simulink model "MicrogridControl"  (R2025b)
settings: Solver=VariableStepAuto  StartTime=0.0  StopTime=8  FixedStep=Ts  RelTol=1e-3
PreLoadFcn:
  | NormalOperation;
  | MicrogridControlParam;
undefined symbols (not defined in the file): base, bessModeInitial, bessSystem, bessVoltage, breakerStatus, DiscIntNeverNeededParam, ee_sli_rtmsupport, event, gcbh, generator, gflInverter, gfmInverter, Inertia, lineInductance, lineResistance, machine, plannedIsland, pmsm, powerLimit, powerQuality, PV, PVInverter, ref, resync, solar, solarInsolationChange, systemFrequency, Ts, windController, windSystem, windTurbine
libraries: nesl_utility x234, ee_lib x174, fl_lib x143, eeGeneralControl x137, simulink x78, eeTransforms x47, slpidlib x23, nesl_utility_internal x12, eePwmGenerator x9, eeSinusoidalMeasurementV2 x9, custom_lib x7, batteryecm_lib x6
(part 15 of 25)

== system MicrogridControl/BESS/BESS Integrated/Detailed/BESS Controller/Grid Forming/VoltageCurrentControl ==
  In Bus Element : Inport  PortName=currentLimiting  Element=Vmd
  In Bus Element1 : Inport  PortName=currentLimiting  Element=Vmq
  In Bus Element6 : Inport  PortName=currentLimiting  Element=Idmax
  In Bus Element7 : Inport  PortName=currentLimiting  Element=Iqmax
  Bus Element In6 : Inport  Port=2  PortName=activeControl  Element=w
  Bus Element In1 : Inport  Port=2  PortName=activeControl  Element=angle
  Reset : Inport  Port=3
  In Bus Element2 : Inport  Port=4  PortName=measure  Element=Vgd
  In Bus Element3 : Inport  Port=4  PortName=measure  Element=Vgq
  In Bus Element4 : Inport  Port=4  PortName=measure  Element=Igd
  In Bus Element5 : Inport  Port=4  PortName=measure  Element=Igq
  Controller : Subsystem
      settings: PortSchema="{\"entries\":[{\"content\":{\"sides\":[{\"content\":{\"connectorIds\":[\"In1\",\"In2\",\"In3\",\"In4\",\"In5\",\"In6\",\"In7\",\"In8\",\"In9\"]},\"type\":\"ConnectorPlacement.EquallySpacedRectSide\",\"uuid\":\"29d30ab3-0ae0-4ae6-aaee-46c6f5faca9c\"},{\"content\":{\"connectorIds\":[\"Out1\",\"Out2\"],\"side\":\"RIGHT\"},\"type\":\"ConnectorPlacement.EquallySpacedRectSide\",\"uuid\":\"4918c3a7-9f8f-4af5-ac25-a0a0710917b2\"},{\"content\":{\"connectorIds\":[\"In10\"],\"side\":\"TOP\"},\"type\":\"ConnectorPlacement.EquallySpacedRectSide\",\"uuid\":\"c6ee8000-0a39-46c2-b8e8-8b73a56a82d9\"}]},\"type\":\"ConnectorPlacement.EquallySpacedConnector\",\"uuid\":\"193e0bc8-3764-41d1-9278-3938c4a9e9f5\"}],\"packageUris\":[\"http://schema.mathworks.com/mf0/Connector/R2020b\"],\"version\":\"1.0\"}"
  Modulation Signal : Subsystem
  mabc : Outport
  wires:
  Reset/1 -> Controller/10(Reset)
  Bus Element In1/1 -> Modulation Signal/3(Angle)
  In Bus Element1/1 -> Controller/3(Vgqref)
  In Bus Element/1 -> Controller/2(Vgdref)
  Bus Element In6/1 -> Controller/1(Angfreq)
  In Bus Element3/1 -> Controller/5(Vsq)
  In Bus Element2/1 -> Controller/4(Vsd)
  In Bus Element7/1 -> Controller/9(Iqmax)
  In Bus Element6/1 -> Controller/8(Idmax)
  In Bus Element5/1 -> Controller/7(Iq)
  In Bus Element4/1 -> Controller/6(Id)
  Controller/1(Vd) -> Modulation Signal/1(Vd)
  Modulation Signal/1(mabc) -> mabc/1
  Controller/2(Vq) -> Modulation Signal/2(Vq)

== system MicrogridControl/BESS/BESS Integrated/Detailed/BESS Plant/Converter/Average ==
  mabc : Inport
  Converter : ee_lib/Semiconductors & Converters/Converters/Average-Value Voltage Source Converter (Three-Phase)  port_option=ee.enum.threePhasePort.composite  frequency_option=ee.enum.converters.frequency.variable  input_option=ee.enum.converters.inputOption.ModWave  FRated=60 Hz  losses_parameterization=ee.enum.converters.losses.fixed  Pfixed=0.5 W  ks=0.01  kc1=1.7 V  kc2=0.01 Ohm  Ploss_vect=[100, 800, 1870, 3250, 4900] W  Irms_vect=[10, 100, 200, 300, 400] A  Vdc_nom=300 V  thermal_mass=30000 J/K  temperature_specify=off  temperature_priority=High  temperature=298.15 K  temperature_nominal_specify=off  temperature_nominal_value=1  temperature_nominal_unit=K
      settings: InternalSimscapePortConfiguration="{\"Bottom\":[],\"Left\":[{\"id\":\"ModWave\",\"label\":\"ModWave\",\"type\":\"input\"},{\"id\":\"N\",\"label\":\"~\",\"type\":\"foundation.electrical.three_phase\"}],\"Right\":[{\"id\":\"p\",\"label\":\"+\",\"type\":\"foundation.electrical.electrical\"},{\"id\":\"n\",\"label\":\"-\",\"type\":\"foundation.electrical.electrical\"}],\"Top\":[]}"
  Simulink-PS Converter : nesl_utility/Simulink-PS Converter  PhysicalDomain=network_engine_domain  SubClassName=ps_input  LeftPortType=input  RightPortType=output  PseudoPeriodic=off  Frequencies=[]  NoiseDistribution=none  NoiseParameters=[]  Unit=1  AffineConversion=off  FilteringAndDerivatives=provide  SimscapeFilterOrder=1  InputFilterTimeConstant=0.001  UdotUserProvided=0
  + : PMIOPort  Side=Left
  - : PMIOPort  Port=2  Side=Left
  ~ : PMIOPort  Port=3  Side=Right
  wires:
  mabc/1 -> Simulink-PS Converter/1
  connections:
  Simulink-PS Converter/RConn1 -- Converter/LConn1
  ~/RConn1 -- Converter/LConn2
  -/RConn1 -- Converter/RConn2
  +/RConn1 -- Converter/RConn1

== system MicrogridControl/BESS/BESS Integrated/Detailed/BESS Plant/Converter/Switching ==
  mabc : Inport
  Add : Sum
  Constant1 : Constant
  Converter : ee_lib/Semiconductors & Converters/Converters/Converter (Three-Phase)  port_option=ee.enum.threePhasePort.composite  fidelity_option=ee.enum.converters.fidelity.detailed  device_type=ee.enum.converters.switchingdevice.ideal  showThermalPort=false  K=0  Vth=1 V  Vgt=1 V  Vgt_off=-1 V  Ih=1 A  Vf=0.8 V  Ron=0.001 Ohm  Rds=0.001 Ohm  Goff=1e-6 1/Ohm  Eon_scalar=22.86e-3 J  Eoff_scalar=17.14e-3 J  Eoff_natural_commutation=10e-3 J  Voff=300 V  Iout_scalar=600 A  onCurrentMeasDelay=0 s  useCurrentFromPreviousCycle=false  useVoltageFromPreviousCycle=false  diode_param=ee.enum.converters.protectiondiode.nodynamics  diode_Vf=0.01 V  diode_Ron=0.0001 Ohm  diode_Goff=1e-5 1/Ohm  diode_C=50 nF  diode_iRM=-235 A  diode_iF=300 A  diode_idot=-50 A/us  diode_trr_param=ee.enum.converters.diodetrr.trr_factor  diode_trr_factor=3  diode_trr=15 us  diode_Qrr=1500 s*uA  diode_rec_loss_model=ee.enum.diode.reverseRecoveryModel.fixed  diode_ErecVal=0 J  diode_scaleWithIandV=false  diode_ErecMat=zeros(2, 3) J  diode_TjrecVec=[298.15, 398.15] K  diode_IfrecVec=[.1, 1, 10] A  diode_IrecVal=10 A  diode_VrecVal=10 V  diode_tFilter=1 / 1000 / 100 s  thermal_network_parameterization=ee.enum.thermalNetworkTopology.external  Rth=[.08, .5] K/W  Rth_Cauer=[.08, .1, .5] K/W  Rth_Foster=[.08, .14, .22, .16] K/W  thermal_mass_parameterization=ee.enum.thermalNetwork.timeconstant  thermal_mass=[.01, .5] J/K  thermal_mass_Cauer=[.01, .1, .5] J/K  thermal_mass_Foster=[.001, .005, .05, .5] J/K  thermal_time_constant=[.001, .2] s  thermal_time_constant_Cauer=[.001, .1, .2] s  thermal_time_constant_Foster=[7e-05, .0007, .01, .08] s  thermal_mass_initial_temperatures=[25, 25] degC  thermal_mass_initial_temperatures_Cauer=[25, 25, 25] degC  junction_thermal_mass=0.01 J/K  Tvec_initial_Foster=[25, 25, 25, 25] degC  snubber_type=ee.enum.converters.snubber.exclude  Cs=1e-7 F  Rs=0.1 Ohm  Vce_loss=[0, 150, 300] V
  Demux : Demux  Outputs=3
  Demux1 : Demux  Outputs=3
  Gain : Gain  Gain=5
  Gain1 : Gain  Gain=0.5
  PWM Generator : eePwmGenerator/PWM Generator  CarrCount=Up  Tper=1/(fSw*1000)  Tdelay=0  Ts=1/(10*fSw*1000)
  Pulse Generation : Subsystem
  Rate Transition1 : RateTransition  OutPortSampleTime=1/(10*fSw*1000)
  Simulink-PS Converter{1..6} (6 alike) : nesl_utility/Simulink-PS Converter  PhysicalDomain=network_engine_domain  SubClassName=ps_input  LeftPortType=input  RightPortType=output  PseudoPeriodic=off  Frequencies=[]  NoiseDistribution=none  NoiseParameters=[]  Unit=1  AffineConversion=off  FilteringAndDerivatives=provide  SimscapeFilterOrder=1  InputFilterTimeConstant=0.001  UdotUserProvided=0
  Six-Pulse Gate Multiplexer : ee_lib/Semiconductors & Converters/Converters/Six-Pulse Gate Multiplexer  port_option=ee.enum.controlport.ps
  + : PMIOPort  Side=Left
  ~ : PMIOPort  Port=2  Side=Right
  - : PMIOPort  Port=3  Side=Left
  wires:
  Demux1/1 -> [AL]
  [BL] -> Simulink-PS Converter3/1
  [AH] -> Simulink-PS Converter6/1
  Demux1/3 -> [CL]
  Gain1/1 -> Rate Transition1/1
  Demux/3 -> [CH]
  Demux/2 -> [BH]
  [CL] -> Simulink-PS Converter1/1
  Constant1/1 -> Add/2
  Add/1 -> Gain1/1
  Gain/1 -> Pulse Generation/1(G)
  PWM Generator/1 -> Gain/1
  mabc/1 -> Add/1
  [CH] -> Simulink-PS Converter2/1
  [AL] -> Simulink-PS Converter5/1
  Demux1/2 -> [BL]
  Demux/1 -> [AH]
  Rate Transition1/1 -> PWM Generator/1
  Pulse Generation/2(G2) -> Demux1/1
  Pulse Generation/1(G1) -> Demux/1
  [BH] -> Simulink-PS Converter4/1
  connections:
  ~/RConn1 -- Converter/LConn2
  Six-Pulse Gate Multiplexer/LConn2 -- Simulink-PS Converter5/RConn1
  Simulink-PS Converter2/RConn1 -- Six-Pulse Gate Multiplexer/LConn5
  Simulink-PS Converter1/RConn1 -- Six-Pulse Gate Multiplexer/LConn6
  Six-Pulse Gate Multiplexer/LConn3 -- Simulink-PS Converter4/RConn1
  Six-Pulse Gate Multiplexer/RConn1 -- Converter/LConn1
  Six-Pulse Gate Multiplexer/LConn1 -- Simulink-PS Converter6/RConn1
  Six-Pulse Gate Multiplexer/LConn4 -- Simulink-PS Converter3/RConn1
  +/RConn1 -- Converter/RConn1
  -/RConn1 -- Converter/RConn2

== system MicrogridControl/BESS/BESS Integrated/Detailed/Filter & Measurements/PLL & Measurements/Measurement1 ==
  u : Inport
  Lead-Lag (Discrete or Continuous) : eeGeneralControl/Lead-Lag (Discrete or Continuous)  T1=0  T2=1e-3  B=inf  A=-inf  init_option=Inherited from block input  x0=0  Ts=Ts
  Vg : Outport
  wires:
  u/1 -> Lead-Lag (Discrete or Continuous)/1
  Lead-Lag (Discrete or Continuous)/1 -> Vg/1

== system MicrogridControl/BESS/BESS Integrated/Detailed/Filter & Measurements/PLL & Measurements/Measurement2 ==
  u : Inport
  Lead-Lag (Discrete or Continuous) : eeGeneralControl/Lead-Lag (Discrete or Continuous)  T1=0  T2=1e-3  B=inf  A=-inf  init_option=Inherited from block input  x0=0  Ts=Ts
  Vg : Outport
  wires:
  u/1 -> Lead-Lag (Discrete or Continuous)/1
  Lead-Lag (Discrete or Continuous)/1 -> Vg/1

== system MicrogridControl/BESS/BESS Integrated/Detailed/Filter & Measurements/PLL & Measurements/Subsystem ==
  Vabc : Inport
  Iabc : Inport  Port=2
  Demux : Demux  Outputs=3
  Demux1 : Demux  Outputs=3
  Park Transform : eeTransforms/Park Transform  AxisAlignment=Q-axis  PowerInvariant=off
  Park Transform1 : eeTransforms/Park Transform  AxisAlignment=Q-axis  PowerInvariant=off
  Scope : Scope  NumInputPorts=2
      settings: ActiveDisplayYMinimum=0.95416  ActiveDisplayYMaximum=1.02793  DataLoggingVariableName=ScopeData5
  Scope1 : Scope  NumInputPorts=2
      settings: ActiveDisplayYMinimum=-2.7903298017751648  ActiveDisplayYMaximum=-1.7770998587100291  DataLoggingVariableName=ScopeData10
  "Sinusoidal Measurement (PLL, Three-Phase)" : eeSinusoidalMeasurementV2/Sinusoidal Measurement (PLL, Three-Phase)  InputFilter=on  InputNormalization=off  Kp_LF=40  Ki_LF=1000  F0=frequency  Theta0=0  Ts=Ts
  Terminator : Terminator
  Terminator1 : Terminator
  mag : Outport
  freq : Outport  Port=2
  angle : Outport  Port=3
  Vd : Outport  Port=4
  Vq : Outport  Port=5
  Id1 : Outport  Port=6
  Iq1 : Outport  Port=7
  wires:
  Iabc/1 -> Park Transform1/1
  Demux1/3 -> Terminator1/1
  Demux1/2 -> Scope1/2, Iq1/1
  Demux1/1 -> Scope1/1, Id1/1
  Park Transform1/1 -> Demux1/1
  "Sinusoidal Measurement (PLL, Three-Phase)"/3 -> mag/1
  "Sinusoidal Measurement (PLL, Three-Phase)"/1 -> freq/1
  "Sinusoidal Measurement (PLL, Three-Phase)"/2 -> Park Transform/2, Park Transform1/2, angle/1
  Demux/2 -> Vq/1, Scope/2
  Demux/1 -> Vd/1, Scope/1
  Park Transform/1 -> Demux/1
  Vabc/1 -> "Sinusoidal Measurement (PLL, Three-Phase)"/1, Park Transform/1
  Demux/3 -> Terminator/1

== system MicrogridControl/BESS/BESS Integrated/Simplified/Grid Forming/Reference Generator/If Action Subsystem ==
  PRef : Inport
  P : Inport  Port=2
  QRef : Inport  Port=3
  Q : Inport  Port=4
  Action Port : ActionPort
  Add : Sum  Inputs=-+
  Add1 : Sum  Inputs=+-
  Add2 : Sum
  Add3 : Sum  Inputs=+-
  Add4 : Sum  Inputs=-+
  Constant : Constant  Value=2*pi*frequency  SampleTime=-1
  Constant2 : Constant
  Constant3 : Constant
  Gain : Gain  Gain=activeDroop
  Gain1 : Gain  Gain=reactiveDroop
  Gain4 : Gain  Gain=Vac
  Gain5 : Gain  Gain=2*pi*frequency
  Integrator with Wrapped State (Discrete or Continuous) : eeGeneralControl/Integrator with Wrapped State (Discrete or Continuous)  LabelModeActiveChoice=Discrete  WrappedStateUpperValue=2*pi  WrappedStateLowerValue=0  x0=0  Ts=-1
  Integrator with Wrapped State (Discrete or Continuous)1 : eeGeneralControl/Integrator with Wrapped State (Discrete or Continuous)  LabelModeActiveChoice=Discrete  WrappedStateUpperValue=2*pi  WrappedStateLowerValue=0  x0=0  Ts=-1
  Saturation : Saturate  UpperLimit=1.1  LowerLimit=0.9
  Scope : Scope
      settings: ActiveDisplayYMinimum=-1  ActiveDisplayYMaximum=1  DataLoggingVariableName=ScopeData2
  Scope1 : Scope
      settings: ActiveDisplayYMinimum=-1  ActiveDisplayYMaximum=1  DataLoggingVariableName=ScopeData3
  Scope2 : Scope  NumInputPorts=2
      settings: ActiveDisplayYMinimum=-1  ActiveDisplayYMaximum=1
  Scope3 : Scope  NumInputPorts=2
      settings: ActiveDisplayYMinimum=-1  ActiveDisplayYMaximum=1  DataLoggingVariableName=ScopeData2
  Vt : Outport
  Ph : Outport  Port=2
  wires:
  Add4/1 -> Scope/1, Gain5/1
  Gain/1 -> Add4/1
  Add1/1 -> Gain1/1
  Add2/1 -> Scope1/1, Saturation/1
  Gain5/1 -> Integrator with Wrapped State (Discrete or Continuous)/1
  Constant3/1 -> Add4/2
  Integrator with Wrapped State (Discrete or Continuous)/1 -> Add3/1
  Constant2/1 -> Add2/2
  Gain1/1 -> Add2/1
  Gain4/1 -> Vt/1
  QRef/1 -> Add1/1, Scope2/1
  Saturation/1 -> Gain4/1
  Add/1 -> Gain/1
  PRef/1 -> Add/1, Scope3/1
  Add3/1 -> Ph/1
  Constant/1 -> Integrator with Wrapped State (Discrete or Continuous)1/1
  Integrator with Wrapped State (Discrete or Continuous)1/1 -> Add3/2
  P/1 -> Add/2, Scope3/2
  Q/1 -> Add1/2, Scope2/2

== system MicrogridControl/BESS/BESS Integrated/Simplified/Grid Forming/Reference Generator/If Action Subsystem1 ==
  PRef : Inport
  P : Inport  Port=2
  VRef : Inport  Port=3
  V : Inport  Port=4
  Action Port : ActionPort
  Add : Sum  Inputs=+-
  Add1 : Sum  Inputs=+-
  Add2 : Sum
  Add3 : Sum  Inputs=+-
  Add4 : Sum  Inputs=-+
  Constant2 : Constant
  Constant3 : Constant
  Constant4 : Constant  Value=0
  Gain : Gain  Gain=reactiveDroop
  Gain1 : Gain  Gain=activeDroop
  Gain4 : Gain  Gain=systemVoltage
  Gain5 : Gain  Gain=2*pi*systemFrequency
  Integrator with Wrapped State (Discrete or Continuous) : eeGeneralControl/Integrator with Wrapped State (Discrete or Continuous)  LabelModeActiveChoice=Discrete  WrappedStateUpperValue=2*pi  WrappedStateLowerValue=0  x0=0  Ts=-1
  Saturation : Saturate  UpperLimit=1.1  LowerLimit=0.9
  Vt : Outport
  Ph : Outport  Port=2
  wires:
  Add/1 -> Gain/1
  Constant4/1 -> Add3/2
  Add4/1 -> Gain5/1
  Gain/1 -> Add4/1
  Add1/1 -> Gain1/1
  Add2/1 -> Saturation/1
  Gain5/1 -> Integrator with Wrapped State (Discrete or Continuous)/1
  Constant3/1 -> Add4/2
  Integrator with Wrapped State (Discrete or Continuous)/1 -> Add3/1
  Constant2/1 -> Add2/2
  Gain1/1 -> Add2/1
  V/1 -> Add/2
  Gain4/1 -> Vt/1
  P/1 -> Add1/2
  VRef/1 -> Add/1
  PRef/1 -> Add1/1
  Add3/1 -> Ph/1
  Saturation/1 -> Gain4/1

== system MicrogridControl/BESS/BESS Integrated1/Detailed/BESS Controller/Grid Following/Current_controller ==
  id-ref : Inport
  ipvd : Inport  Port=2
  iqref : Inport  Port=3
  iq : Inport  Port=4
  Vd : Inport  Port=5
  Vq : Inport  Port=6
  Constant4 : Constant  Value=0
  Gain1 : Gain  Gain=2*1*pi*frequency*L/zbase
  Gain2 : Gain  Gain=2*1*pi*frequency*L/zbase
  Mux1 : Mux  Inputs=3
  PID Controller : slpidlib/PID Controller  Controller=PID  Form=Parallel  TimeDomain=Discrete-time  UseExternalTs=off  SampleTime=-1  IntegratorMethod=Forward Euler  FilterMethod=Forward Euler  ControllerParametersSource=internal  P=Kpic  I=Kiic  UseKiTs=off  D=Kd  UseExternalDerivativeSource=off  N=100  UseFilter=on  TunerSelectOption=Transfer Function Based (PID Tuner App)  InitialConditionSource=internal  InitialConditionForIntegrator=0  InitialConditionForFilter=0  DifferentiatorICPrevScaledInput=0  ExternalReset=none  TrackingMode=off  Kt=1  LimitOutput=off  SatLimitsSource=internal  UpperSaturationLimit=inf  LowerSaturationLimit=-inf  LinearizeAsGain=on  AntiWindupMode=none  Kb=1  LimitIntegrator=off  UpperIntegratorSaturationLimit=inf  LowerIntegratorSaturationLimit=-inf  POutMin=[]  POutMax=[]  IOutMin=[]  IOutMax=[]  DOutMin=[]  DOutMax=[]  NOutMin=[]  NOutMax=[]  SumOutMin=[]  SumOutMax=[]  SaturationOutMin=[]  SaturationOutMax=[]  PParamMin=[]  PParamMax=[]  IParamMin=[]  IParamMax=[]  DParamMin=[]  DParamMax=[]  NParamMin=[]  NParamMax=[]  KbParamMin=[]  KbParamMax=[]  KtParamMin=[]  KtParamMax=[]  KbOutMin=[]  KbOutMax=[]  KtOutMin=[]  KtOutMax=[]  IntegratorOutMin=[]  IntegratorOutMax=[]  FilterOutMin=[]  FilterOutMax=[]  SumI1OutMin=[]  SumI1OutMax=[]  SumI2OutMin=[]  SumI2OutMax=[]  SumI3OutMin=[]  SumI3OutMax=[]  SumI4OutMin=[]  SumI4OutMax=[]  SumDOutMin=[]  SumDOutMax=[]  DifferentiatorOutMin=[]  DifferentiatorOutMax=[]  FilterDiffOutCoefMin=[]  FilterDiffOutCoefMax=[]  ReciprocalOutMin=[]  ReciprocalOutMax=[]  SumDenOutMin=[]  SumDenOutMax=[]  SumNumOutMin=[]  SumNumOutMax=[]  DivideOutMin=[]  DivideOutMax=[]  UdiffTsProdOutMin=[]  UdiffTsProdOutMax=[]  NTsProdOutMin=[]  NTsProdOutMax=[]  UintegralTsProdOutMin=[]  UintegralTsProdOutMax=[]  UngainTsProdOutMin=[]  UngainTsProdOutMax=[]  ClampingZeroOutDataTypeStr=Inherit: Inherit via back propagation  ClampingZeroOutMin=[]  ClampingZeroOutMax=[]  FilterDenConstantOutDataTypeStr=Inherit: Inherit via back propagation  FilterDenConstantOutMin=[]  FilterDenConstantOutMax=[]  PCopyOutDataTypeStr=Inherit: Inherit via back propagation  PCopyOutMin=[]  PCopyOutMax=[]  NCopyOutDataTypeStr=Inherit: Inherit via back propagation  NCopyOutMin=[]  NCopyOutMax=[]  IntegratorContinuousStateAttributes=''  IntegratorStateMustResolveToSignalObject=off  IntegratorRTWStateStorageClass=Auto  FilterContinuousStateAttributes=''  FilterStateMustResolveToSignalObject=off  FilterRTWStateStorageClass=Auto  ParallelPVariant=InternalParameters  IdealPVariant=Disabled  IVariant=InternalParameters  DVariant=InternalParameters  IntegratorVariant=Discrete  SatVariant=Disabled  AWVariant=Passthrough  PCopyVariant=Disabled  TRVariant=Disabled  FdbkBlocksVariant=Forward  IdealPFdbkVariant=Disabled  SatFdbkVariant=Disabled  DerivativeFilterVariant=ForwardEulerFilter  NVariant=InternalParameters  NCopyVariant=Disabled  FilterICVariant=InternalICsFilter  IntegratorICVariant=InternalICs  ExternalResetVariant=Disabled  TRSumVariant=Passthrough  SumFdbkVariant=Disabled  SumVariant=Sum_PID  TsampFilterVariant=InternalTs  TsampNgainVariant=Passthrough  TsampIntegralVariant=Disabled_SignalSpec  ExternalSaturationOutDataTypeStr=Inherit: Same as second input  DerivativeSourceVariant=ErrorSignal  PreIntVariant=InternalPreInt
  PID Controller1 : slpidlib/PID Controller  Controller=PID  Form=Parallel  TimeDomain=Discrete-time  UseExternalTs=off  SampleTime=-1  IntegratorMethod=Forward Euler  FilterMethod=Forward Euler  ControllerParametersSource=internal  P=Kpic  I=Kiic  UseKiTs=off  D=Kd  UseExternalDerivativeSource=off  N=100  UseFilter=on  TunerSelectOption=Transfer Function Based (PID Tuner App)  InitialConditionSource=internal  InitialConditionForIntegrator=0  InitialConditionForFilter=0  DifferentiatorICPrevScaledInput=0  ExternalReset=none  TrackingMode=off  Kt=1  LimitOutput=off  SatLimitsSource=internal  UpperSaturationLimit=inf  LowerSaturationLimit=-inf  LinearizeAsGain=on  AntiWindupMode=none  Kb=1  LimitIntegrator=off  UpperIntegratorSaturationLimit=inf  LowerIntegratorSaturationLimit=-inf  POutMin=[]  POutMax=[]  IOutMin=[]  IOutMax=[]  DOutMin=[]  DOutMax=[]  NOutMin=[]  NOutMax=[]  SumOutMin=[]  SumOutMax=[]  SaturationOutMin=[]  SaturationOutMax=[]  PParamMin=[]  PParamMax=[]  IParamMin=[]  IParamMax=[]  DParamMin=[]  DParamMax=[]  NParamMin=[]  NParamMax=[]  KbParamMin=[]  KbParamMax=[]  KtParamMin=[]  KtParamMax=[]  KbOutMin=[]  KbOutMax=[]  KtOutMin=[]  KtOutMax=[]  IntegratorOutMin=[]  IntegratorOutMax=[]  FilterOutMin=[]  FilterOutMax=[]  SumI1OutMin=[]  SumI1OutMax=[]  SumI2OutMin=[]  SumI2OutMax=[]  SumI3OutMin=[]  SumI3OutMax=[]  SumI4OutMin=[]  SumI4OutMax=[]  SumDOutMin=[]  SumDOutMax=[]  DifferentiatorOutMin=[]  DifferentiatorOutMax=[]  FilterDiffOutCoefMin=[]  FilterDiffOutCoefMax=[]  ReciprocalOutMin=[]  ReciprocalOutMax=[]  SumDenOutMin=[]  SumDenOutMax=[]  SumNumOutMin=[]  SumNumOutMax=[]  DivideOutMin=[]  DivideOutMax=[]  UdiffTsProdOutMin=[]  UdiffTsProdOutMax=[]  NTsProdOutMin=[]  NTsProdOutMax=[]  UintegralTsProdOutMin=[]  UintegralTsProdOutMax=[]  UngainTsProdOutMin=[]  UngainTsProdOutMax=[]  ClampingZeroOutDataTypeStr=Inherit: Inherit via back propagation  ClampingZeroOutMin=[]  ClampingZeroOutMax=[]  FilterDenConstantOutDataTypeStr=Inherit: Inherit via back propagation  FilterDenConstantOutMin=[]  FilterDenConstantOutMax=[]  PCopyOutDataTypeStr=Inherit: Inherit via back propagation  PCopyOutMin=[]  PCopyOutMax=[]  NCopyOutDataTypeStr=Inherit: Inherit via back propagation  NCopyOutMin=[]  NCopyOutMax=[]  IntegratorContinuousStateAttributes=''  IntegratorStateMustResolveToSignalObject=off  IntegratorRTWStateStorageClass=Auto  FilterContinuousStateAttributes=''  FilterStateMustResolveToSignalObject=off  FilterRTWStateStorageClass=Auto  ParallelPVariant=InternalParameters  IdealPVariant=Disabled  IVariant=InternalParameters  DVariant=InternalParameters  IntegratorVariant=Discrete  SatVariant=Disabled  AWVariant=Passthrough  PCopyVariant=Disabled  TRVariant=Disabled  FdbkBlocksVariant=Forward  IdealPFdbkVariant=Disabled  SatFdbkVariant=Disabled  DerivativeFilterVariant=ForwardEulerFilter  NVariant=InternalParameters  NCopyVariant=Disabled  FilterICVariant=InternalICsFilter  IntegratorICVariant=InternalICs  ExternalResetVariant=Disabled  TRSumVariant=Passthrough  SumFdbkVariant=Disabled  SumVariant=Sum_PID  TsampFilterVariant=InternalTs  TsampNgainVariant=Passthrough  TsampIntegralVariant=Disabled_SignalSpec  ExternalSaturationOutDataTypeStr=Inherit: Same as second input  DerivativeSourceVariant=ErrorSignal  PreIntVariant=InternalPreInt
  Scope : Scope  NumInputPorts=2
      settings: ActiveDisplayYMinimum=-1  ActiveDisplayYMaximum=1
  Scope1 : Scope  NumInputPorts=2
      settings: ActiveDisplayYMinimum=-1.21282  ActiveDisplayYMaximum=0.9154  DataLoggingVariableName=ScopeData2
  Sum1 : Sum  Inputs=|+-
  Sum3 : Sum  Inputs=|++-
  Sum4 : Sum  Inputs=|+++
  Sum5 : Sum  Inputs=|+-
  mdq0 : Outport
  wires:
  iqref/1 -> Sum5/1, Scope1/1
  Mux1/1 -> mdq0/1
  Sum4/1 -> [Eq], Mux1/2
  PID Controller1/1 -> Sum4/1
  Sum5/1 -> PID Controller1/1
  Constant4/1 -> Mux1/3
  Vd/1 -> Sum3/1
  Sum1/1 -> PID Controller/1
  iq/1 -> Sum5/2, Gain2/1, Scope1/2
  Vq/1 -> Sum4/2
  Gain1/1 -> Sum4/3
  id-ref/1 -> Sum1/1, Scope/1
  ipvd/1 -> Sum1/2, Gain1/1, Scope/2
  Gain2/1 -> Sum3/3
  Sum3/1 -> [Ed], Mux1/1
  PID Controller/1 -> Sum3/2

== system MicrogridControl/BESS/BESS Integrated1/Detailed/BESS Controller/Grid Following/Reference Current ==
  note: Avoid division by zero during start
  note: Current Limiters
  V_ref : Inport
  V-mag : Inport  Port=2
  del f : Inport  Port=3
  LVRT_iq : Inport  Port=4
  PRef : Inport  Port=5
  QRef : Inport  Port=6
  Constant1 : Constant
  Constant3 : Constant  Value=Imax
  Current limits : Subsystem
  Refernce id generation : Subsystem
  Refernce iq generation : Subsystem
  Switch : Switch  Criteria=u2 ~= 0  SaturateOnIntegerOverflow=off  InputSameDT=off
  Unit Delay1 : UnitDelay  SampleTime=Ts  HasFrameUpgradeWarning=on
  Unit Delay3 : UnitDelay  SampleTime=Ts  HasFrameUpgradeWarning=on
  id_ref : Outport
  iq_ref : Outport  Port=2
  wires:
  Current limits/2(iubd) -> Refernce id generation/3(ubid)
  PRef/1 -> Refernce id generation/4(PRef)
  QRef/1 -> Refernce iq generation/5(Q_ref)
  Constant1/1 -> Switch/3
  Switch/1 -> Refernce iq generation/3(V_mag), Refernce id generation/1(V_mag)
  V-mag/1 -> Switch/2, Switch/1
  LVRT_iq/1 -> Refernce iq generation/4(LVRT_iq)
  Refernce iq generation/1(iq_ref) -> iq_ref/1, Unit Delay1/1
  V_ref/1 -> Refernce iq generation/2(V_ref)
  del f/1 -> Refernce id generation/2(del f)
  Refernce id generation/1(id_ref) -> Unit Delay3/1, id_ref/1
  Constant3/1 -> Current limits/1(Imax)
  Unit Delay3/1 -> Current limits/3(idref)
  Current limits/1(iubq) -> Refernce iq generation/1(ubiq)
  Unit Delay1/1 -> Current limits/2(iqref)

== system MicrogridControl/BESS/BESS Integrated1/Detailed/BESS Controller/Grid Forming/Current Limiting ==
  In Bus Element : Inport  PortName=measure  Element=Igd
  In Bus Element1 : Inport  PortName=measure  Element=Igq
  In Bus Element2 : Inport  Port=2  PortName=reactiveControl  Element=Vmd
  In Bus Element4 : Inport  Port=2  PortName=reactiveControl  Element=Vmq
  CurrentLimitingMethod : Subsystem  Variant=on  VariantControlMode=label  VariantControl=Choice  LabelModeActiveChoice=ctSat
  Scope : Scope  NumInputPorts=2
  Subtract : Sum  Inputs=+-
  Subtract1 : Sum  Inputs=-+
  Out Bus Element : Outport  PortName=currentLimiting  Element=Vmd
  Out Bus Element1 : Outport  PortName=currentLimiting  Element=Vmq
  Out Bus Element2 : Outport  PortName=currentLimiting  Element=Idmax
  Out Bus Element3 : Outport  PortName=currentLimiting  Element=Iqmax
  wires:
  CurrentLimitingMethod/2(delVq) -> Subtract1/1
  CurrentLimitingMethod/1(delVd) -> Subtract/2
  CurrentLimitingMethod/3(Idmax) -> Out Bus Element2/1
  In Bus Element/1 -> CurrentLimitingMethod/1(Igd)  "Q"
  CurrentLimitingMethod/4(Iqmax) -> Out Bus Element3/1
  Subtract1/1 -> Out Bus Element1/1, Scope/2
  Subtract/1 -> Out Bus Element/1, Scope/1
  In Bus Element4/1 -> Subtract1/2
  In Bus Element1/1 -> CurrentLimitingMethod/2(Igq)
  In Bus Element2/1 -> Subtract/1

== system MicrogridControl/BESS/BESS Integrated1/Detailed/BESS Controller/Grid Forming/Grid Voltage Reactive Power Support ==
  In Bus Element1 : Inport  PortName=measure  Element=Vgd
  In Bus Element3 : Inport  PortName=measure  Element=Vgq
  In Bus Element2 : Inport  PortName=measure  Element=Igd
  In Bus Element4 : Inport  PortName=measure  Element=Igq
  PrefInput : Inport  Port=2
  QrefInput : Inport  Port=3
  Modifying Active Power Reference : Subsystem
  Modifying Reactive Power Reference : Subsystem
  Scope : Scope
  Scope1 : Scope
      settings: ActiveDisplayYMinimum=0.9  ActiveDisplayYMaximum=1.1
  Scope2 : Scope
      settings: ActiveDisplayYMinimum=-1  ActiveDisplayYMaximum=1
  Pref : Outport
  Qref : Outport  Port=2
  wires:
  Modifying Reactive Power Reference/2(QrefNew) -> Qref/1, Scope2/1
  Modifying Reactive Power Reference/1(PrefNew) -> Pref/1, Scope1/1
  QrefInput/1 -> Modifying Reactive Power Reference/3(Qref)
  In Bus Element3/1 -> Modifying Reactive Power Reference/2(Vgq)
  In Bus Element1/1 -> Modifying Active Power Reference/2(Vd), Modifying Reactive Power Reference/1(Vgd)
  In Bus Element4/1 -> Modifying Active Power Reference/4(Igq)
  In Bus Element2/1 -> Modifying Active Power Reference/3(Igd)
  PrefInput/1 -> Modifying Active Power Reference/1(PrefInput)
  Modifying Active Power Reference/1(Pref) -> Modifying Reactive Power Reference/4(Pref), Scope/1

== system MicrogridControl/BESS/BESS Integrated1/Detailed/BESS Controller/Grid Forming/Measurement ==
  Vgabcc : Inport
  Igabc : Inport  Port=2
  Angle : Inport  Port=3
  Frequency Measurement : Subsystem
  Gain1 : Gain  Gain=2/3
  Gain2 : Gain  Gain=2/3
  Gain3 : Gain  Gain=1%/(girdLineVoltage*sqrt(2/3))
  Gain4 : Gain  Gain=1%/(girdLineVoltage*sqrt(2/3))
  Gain5 : Gain  Gain=1%/(power/(sqrt(3)*girdLineVoltage)*sqrt(2))
  Gain6 : Gain  Gain=1%/(power/(sqrt(3)*girdLineVoltage)*sqrt(2))
  Power Measurement (Three-Phase) : eePowerMeasurement/Power Measurement (Three-Phase)  LabelModeActiveChoice=Discrete  F=powerFreq  K=[1]  Seq=Positive  Ts=measSampleTime
  abc2dq : Subsystem
  Out Bus Element : Outport  PortName=measure  Element=P
  Out Bus Element1 : Outport  PortName=measure  Element=Q
  Out Bus Element2 : Outport  PortName=measure  Element=Vgd
  Out Bus Element3 : Outport  PortName=measure  Element=Vgq
  Out Bus Element4 : Outport  PortName=measure  Element=Igd
  Out Bus Element5 : Outport  PortName=measure  Element=Igq
  Out Bus Element6 : Outport  PortName=measure  Element=fgrid
  Pmeas : Outport  Port=2
  Qmeas : Outport  Port=3
  fmeas : Outport  Port=4
  wires:
  Frequency Measurement/1(freq) -> fmeas/1, Out Bus Element6/1
  Gain6/1 -> Out Bus Element5/1  "Igq"
  Gain5/1 -> Out Bus Element4/1  "Igd"
  Gain4/1 -> Out Bus Element2/1  "Vgd"
  Gain3/1 -> Out Bus Element3/1  "Vgq"
  abc2dq/4(Igq) -> Gain6/1
  abc2dq/3(Igd) -> Gain5/1
  abc2dq/2(Vgq) -> Gain3/1
  abc2dq/1(Vgd) -> Gain4/1
  Gain1/1 -> Out Bus Element1/1, Qmeas/1  "Qmeas"
  Gain2/1 -> Out Bus Element/1, Pmeas/1  "Pmeas"
  Power Measurement (Three-Phase)/2 -> Gain1/1
  Igabc/1 -> Power Measurement (Three-Phase)/2, abc2dq/1(Igabc)  "Iabc"
  Power Measurement (Three-Phase)/1 -> Gain2/1
  Angle/1 -> abc2dq/2(Angle)
  Vgabcc/1 -> Power Measurement (Three-Phase)/1, Frequency Measurement/1(Vabc), abc2dq/3(Vgabc)  "Vabc"

== system MicrogridControl/BESS/BESS Integrated1/Detailed/BESS Controller/Grid Forming/Power Control ==
  note: Active Power Control
  note: Reactive Power Control
  In Bus Element2 : Inport  PortName=measure  Element=P
  In Bus Element1 : Inport  PortName=measure  Element=fgrid
  BusElementIn : Inport  PortName=measure  Element=Vgd
  BusElementIn2 : Inport  PortName=measure  Element=Q
  Pref : Inport  Port=2
  Qref : Inport  Port=3
  Vref : Inport  Port=4
  Fref : Inport  Port=5
  CntrlFlag : Inport  Port=6
  ActivePowerControl : Subsystem  Variant=on  VariantControlMode=label  VariantControl=Choice  LabelModeActiveChoice=vsm
  ReactiveControl : Subsystem
  Scope : Scope
      settings: ActiveDisplayYMinimum=-13.20558  ActiveDisplayYMaximum=19.03908  DataLoggingVariableName=ScopeData16
  Out Bus Element : Outport  PortName=reactiveControl  Element=Vmd
  Out Bus Element1 : Outport  PortName=reactiveControl  Element=Vmq
  Out Bus Element6 : Outport  Port=2  PortName=activeControl  Element=angle
  Out Bus Element4 : Outport  Port=2  PortName=activeControl  Element=w
  angle : Outport  Port=3
  wires:
  BusElementIn2/1 -> ReactiveControl/3(Qmeas)
  BusElementIn/1 -> ReactiveControl/4(Vgdmeas), Scope/1
  [Cntrlflag] -> ReactiveControl/1(CntrlFlag)
  Vref/1 -> ReactiveControl/5(Vref)
  [Cntrlflag] -> ActivePowerControl/4(cntrlflag)
  CntrlFlag/1 -> [Cntrlflag]
  Fref/1 -> ActivePowerControl/3(fref)
  In Bus Element1/1 -> ActivePowerControl/5(fgrid)
  In Bus Element2/1 -> ActivePowerControl/2(Pmeas)
  Qref/1 -> ReactiveControl/2(Qref)  "Q"
  Pref/1 -> ActivePowerControl/1(Pref)  "Q"
  ReactiveControl/2(Vmq) -> Out Bus Element1/1
  ReactiveControl/1(Vmd) -> Out Bus Element/1
  ActivePowerControl/1(Theta) -> Out Bus Element6/1, angle/1
  ActivePowerControl/2(w) -> Out Bus Element4/1

== system MicrogridControl/BESS/BESS Integrated1/Detailed/BESS Controller/Grid Forming/Subsystem2 ==
  In : Inport
  Reset : Inport  Port=2
  AND : Logic  IconShape=distinctive  AllPortsSameDT=off  OutDataTypeStr=boolean
  Data Type Conversion : DataTypeConversion  SaturateOnIntegerOverflow=off  RndMeth=Floor
  Delay : Delay  DelayLength=1  SampleTime=Ts*20000
  Delay1 : Delay  DelayLength=1
  NOT : Logic  Operator=NOT  IconShape=distinctive  AllPortsSameDT=off  OutDataTypeStr=boolean
  NOT1 : Logic  Operator=NOT  IconShape=distinctive  AllPortsSameDT=off  OutDataTypeStr=boolean
  Product : Product
  mabc : Outport
  wires:
  In/1 -> Product/2
  Reset/1 -> AND/1, Delay/1
  NOT/1 -> AND/2
  Delay/1 -> NOT/1
  Product/1 -> Delay1/1
  AND/1 -> NOT1/1
  NOT1/1 -> Data Type Conversion/1
  Data Type Conversion/1 -> Product/1
  Delay1/1 -> mabc/1

== system MicrogridControl/BESS/BESS Integrated1/Detailed/BESS Controller/Grid Forming/VoltageCurrentControl ==
  In Bus Element : Inport  PortName=currentLimiting  Element=Vmd
  In Bus Element1 : Inport  PortName=currentLimiting  Element=Vmq
  In Bus Element6 : Inport  PortName=currentLimiting  Element=Idmax
  In Bus Element7 : Inport  PortName=currentLimiting  Element=Iqmax
  Bus Element In6 : Inport  Port=2  PortName=activeControl  Element=w
  Bus Element In1 : Inport  Port=2  PortName=activeControl  Element=angle
  Reset : Inport  Port=3
  In Bus Element2 : Inport  Port=4  PortName=measure  Element=Vgd
  In Bus Element3 : Inport  Port=4  PortName=measure  Element=Vgq
  In Bus Element4 : Inport  Port=4  PortName=measure  Element=Igd
  In Bus Element5 : Inport  Port=4  PortName=measure  Element=Igq
  Controller : Subsystem
      settings: PortSchema="{\"entries\":[{\"content\":{\"sides\":[{\"content\":{\"connectorIds\":[\"In1\",\"In2\",\"In3\",\"In4\",\"In5\",\"In6\",\"In7\",\"In8\",\"In9\"]},\"type\":\"ConnectorPlacement.EquallySpacedRectSide\",\"uuid\":\"29d30ab3-0ae0-4ae6-aaee-46c6f5faca9c\"},{\"content\":{\"connectorIds\":[\"Out1\",\"Out2\"],\"side\":\"RIGHT\"},\"type\":\"ConnectorPlacement.EquallySpacedRectSide\",\"uuid\":\"4918c3a7-9f8f-4af5-ac25-a0a0710917b2\"},{\"content\":{\"connectorIds\":[\"In10\"],\"side\":\"TOP\"},\"type\":\"ConnectorPlacement.EquallySpacedRectSide\",\"uuid\":\"c6ee8000-0a39-46c2-b8e8-8b73a56a82d9\"}]},\"type\":\"ConnectorPlacement.EquallySpacedConnector\",\"uuid\":\"193e0bc8-3764-41d1-9278-3938c4a9e9f5\"}],\"packageUris\":[\"http://schema.mathworks.com/mf0/Connector/R2020b\"],\"version\":\"1.0\"}"
  Modulation Signal : Subsystem
  mabc : Outport
  wires:
  Reset/1 -> Controller/10(Reset)
  Bus Element In1/1 -> Modulation Signal/3(Angle)
  In Bus Element1/1 -> Controller/3(Vgqref)
  In Bus Element/1 -> Controller/2(Vgdref)
  Bus Element In6/1 -> Controller/1(Angfreq)
  In Bus Element3/1 -> Controller/5(Vsq)
  In Bus Element2/1 -> Controller/4(Vsd)
  In Bus Element7/1 -> Controller/9(Iqmax)
  In Bus Element6/1 -> Controller/8(Idmax)
  In Bus Element5/1 -> Controller/7(Iq)
  In Bus Element4/1 -> Controller/6(Id)
  Controller/1(Vd) -> Modulation Signal/1(Vd)
  Modulation Signal/1(mabc) -> mabc/1
  Controller/2(Vq) -> Modulation Signal/2(Vq)

== system MicrogridControl/BESS/BESS Integrated1/Detailed/BESS Plant/Converter/Average ==
  mabc : Inport
  Converter : ee_lib/Semiconductors & Converters/Converters/Average-Value Voltage Source Converter (Three-Phase)  port_option=ee.enum.threePhasePort.composite  frequency_option=ee.enum.converters.frequency.variable  input_option=ee.enum.converters.inputOption.ModWave  FRated=60 Hz  losses_parameterization=ee.enum.converters.losses.fixed  Pfixed=0.5 W  ks=0.01  kc1=1.7 V  kc2=0.01 Ohm  Ploss_vect=[100, 800, 1870, 3250, 4900] W  Irms_vect=[10, 100, 200, 300, 400] A  Vdc_nom=300 V  thermal_mass=30000 J/K  temperature_specify=off  temperature_priority=High  temperature=298.15 K  temperature_nominal_specify=off  temperature_nominal_value=1  temperature_nominal_unit=K
      settings: InternalSimscapePortConfiguration="{\"Bottom\":[],\"Left\":[{\"id\":\"ModWave\",\"label\":\"ModWave\",\"type\":\"input\"},{\"id\":\"N\",\"label\":\"~\",\"type\":\"foundation.electrical.three_phase\"}],\"Right\":[{\"id\":\"p\",\"label\":\"+\",\"type\":\"foundation.electrical.electrical\"},{\"id\":\"n\",\"label\":\"-\",\"type\":\"foundation.electrical.electrical\"}],\"Top\":[]}"
  Simulink-PS Converter : nesl_utility/Simulink-PS Converter  PhysicalDomain=network_engine_domain  SubClassName=ps_input  LeftPortType=input  RightPortType=output  PseudoPeriodic=off  Frequencies=[]  NoiseDistribution=none  NoiseParameters=[]  Unit=1  AffineConversion=off  FilteringAndDerivatives=provide  SimscapeFilterOrder=1  InputFilterTimeConstant=0.001  UdotUserProvided=0
  + : PMIOPort  Side=Left
  - : PMIOPort  Port=2  Side=Left
  ~ : PMIOPort  Port=3  Side=Right
  wires:
  mabc/1 -> Simulink-PS Converter/1
  connections:
  Simulink-PS Converter/RConn1 -- Converter/LConn1
  ~/RConn1 -- Converter/LConn2
  -/RConn1 -- Converter/RConn2
  +/RConn1 -- Converter/RConn1

== system MicrogridControl/BESS/BESS Integrated1/Detailed/BESS Plant/Converter/Switching ==
  mabc : Inport
  Add : Sum
  Constant1 : Constant
  Converter : ee_lib/Semiconductors & Converters/Converters/Converter (Three-Phase)  port_option=ee.enum.threePhasePort.composite  fidelity_option=ee.enum.converters.fidelity.detailed  device_type=ee.enum.converters.switchingdevice.ideal  showThermalPort=false  K=0  Vth=1 V  Vgt=1 V  Vgt_off=-1 V  Ih=1 A  Vf=0.8 V  Ron=0.001 Ohm  Rds=0.001 Ohm  Goff=1e-6 1/Ohm  Eon_scalar=22.86e-3 J  Eoff_scalar=17.14e-3 J  Eoff_natural_commutation=10e-3 J  Voff=300 V  Iout_scalar=600 A  onCurrentMeasDelay=0 s  useCurrentFromPreviousCycle=false  useVoltageFromPreviousCycle=false  diode_param=ee.enum.converters.protectiondiode.nodynamics  diode_Vf=0.01 V  diode_Ron=0.0001 Ohm  diode_Goff=1e-5 1/Ohm  diode_C=50 nF  diode_iRM=-235 A  diode_iF=300 A  diode_idot=-50 A/us  diode_trr_param=ee.enum.converters.diodetrr.trr_factor  diode_trr_factor=3  diode_trr=15 us  diode_Qrr=1500 s*uA  diode_rec_loss_model=ee.enum.diode.reverseRecoveryModel.fixed  diode_ErecVal=0 J  diode_scaleWithIandV=false  diode_ErecMat=zeros(2, 3) J  diode_TjrecVec=[298.15, 398.15] K  diode_IfrecVec=[.1, 1, 10] A  diode_IrecVal=10 A  diode_VrecVal=10 V  diode_tFilter=1 / 1000 / 100 s  thermal_network_parameterization=ee.enum.thermalNetworkTopology.external  Rth=[.08, .5] K/W  Rth_Cauer=[.08, .1, .5] K/W  Rth_Foster=[.08, .14, .22, .16] K/W  thermal_mass_parameterization=ee.enum.thermalNetwork.timeconstant  thermal_mass=[.01, .5] J/K  thermal_mass_Cauer=[.01, .1, .5] J/K  thermal_mass_Foster=[.001, .005, .05, .5] J/K  thermal_time_constant=[.001, .2] s  thermal_time_constant_Cauer=[.001, .1, .2] s  thermal_time_constant_Foster=[7e-05, .0007, .01, .08] s  thermal_mass_initial_temperatures=[25, 25] degC  thermal_mass_initial_temperatures_Cauer=[25, 25, 25] degC  junction_thermal_mass=0.01 J/K  Tvec_initial_Foster=[25, 25, 25, 25] degC  snubber_type=ee.enum.converters.snubber.exclude  Cs=1e-7 F  Rs=0.1 Ohm  Vce_loss=[0, 150, 300] V
  Demux : Demux  Outputs=3
  Demux1 : Demux  Outputs=3
  Gain : Gain  Gain=5
  Gain1 : Gain  Gain=0.5
  PWM Generator : eePwmGenerator/PWM Generator  CarrCount=Up  Tper=1/(fSw*1000)  Tdelay=0  Ts=1/(10*fSw*1000)
  Pulse Generation : Subsystem
  Rate Transition1 : RateTransition  OutPortSampleTime=1/(10*fSw*1000)
  Simulink-PS Converter{1..6} (6 alike) : nesl_utility/Simulink-PS Converter  PhysicalDomain=network_engine_domain  SubClassName=ps_input  LeftPortType=input  RightPortType=output  PseudoPeriodic=off  Frequencies=[]  NoiseDistribution=none  NoiseParameters=[]  Unit=1  AffineConversion=off  FilteringAndDerivatives=provide  SimscapeFilterOrder=1  InputFilterTimeConstant=0.001  UdotUserProvided=0
  Six-Pulse Gate Multiplexer : ee_lib/Semiconductors & Converters/Converters/Six-Pulse Gate Multiplexer  port_option=ee.enum.controlport.ps
  + : PMIOPort  Side=Left
  ~ : PMIOPort  Port=2  Side=Right
  - : PMIOPort  Port=3  Side=Left
  wires:
  Demux1/1 -> [AL]
  [BL] -> Simulink-PS Converter3/1
  [AH] -> Simulink-PS Converter6/1
  Demux1/3 -> [CL]
  Gain1/1 -> Rate Transition1/1
  Demux/3 -> [CH]
  Demux/2 -> [BH]
  [CL] -> Simulink-PS Converter1/1
  Constant1/1 -> Add/2
  Add/1 -> Gain1/1
  Gain/1 -> Pulse Generation/1(G)
  PWM Generator/1 -> Gain/1
  mabc/1 -> Add/1
  [CH] -> Simulink-PS Converter2/1
  [AL] -> Simulink-PS Converter5/1
  Demux1/2 -> [BL]
  Demux/1 -> [AH]
  Rate Transition1/1 -> PWM Generator/1
  Pulse Generation/2(G2) -> Demux1/1
  Pulse Generation/1(G1) -> Demux/1
  [BH] -> Simulink-PS Converter4/1
  connections:
  ~/RConn1 -- Converter/LConn2
  Six-Pulse Gate Multiplexer/LConn2 -- Simulink-PS Converter5/RConn1
  Simulink-PS Converter2/RConn1 -- Six-Pulse Gate Multiplexer/LConn5
  Simulink-PS Converter1/RConn1 -- Six-Pulse Gate Multiplexer/LConn6
  Six-Pulse Gate Multiplexer/LConn3 -- Simulink-PS Converter4/RConn1
  Six-Pulse Gate Multiplexer/RConn1 -- Converter/LConn1
  Six-Pulse Gate Multiplexer/LConn1 -- Simulink-PS Converter6/RConn1
  Six-Pulse Gate Multiplexer/LConn4 -- Simulink-PS Converter3/RConn1
  +/RConn1 -- Converter/RConn1
  -/RConn1 -- Converter/RConn2

== system MicrogridControl/BESS/BESS Integrated1/Detailed/Filter & Measurements/PLL & Measurements/Measurement1 ==
  u : Inport
  Lead-Lag (Discrete or Continuous) : eeGeneralControl/Lead-Lag (Discrete or Continuous)  T1=0  T2=1e-3  B=inf  A=-inf  init_option=Inherited from block input  x0=0  Ts=Ts
  Vg : Outport
  wires:
  u/1 -> Lead-Lag (Discrete or Continuous)/1
  Lead-Lag (Discrete or Continuous)/1 -> Vg/1

== system MicrogridControl/BESS/BESS Integrated1/Detailed/Filter & Measurements/PLL & Measurements/Measurement2 ==
  u : Inport
  Lead-Lag (Discrete or Continuous) : eeGeneralControl/Lead-Lag (Discrete or Continuous)  T1=0  T2=1e-3  B=inf  A=-inf  init_option=Inherited from block input  x0=0  Ts=Ts
  Vg : Outport
  wires:
  u/1 -> Lead-Lag (Discrete or Continuous)/1
  Lead-Lag (Discrete or Continuous)/1 -> Vg/1

== system MicrogridControl/BESS/BESS Integrated1/Detailed/Filter & Measurements/PLL & Measurements/Subsystem ==
  Vabc : Inport
  Iabc : Inport  Port=2
  Demux : Demux  Outputs=3
  Demux1 : Demux  Outputs=3
  Park Transform : eeTransforms/Park Transform  AxisAlignment=Q-axis  PowerInvariant=off
  Park Transform1 : eeTransforms/Park Transform  AxisAlignment=Q-axis  PowerInvariant=off
  Scope : Scope  NumInputPorts=2
      settings: ActiveDisplayYMinimum=0.95416  ActiveDisplayYMaximum=1.02793  DataLoggingVariableName=ScopeData5
  Scope1 : Scope  NumInputPorts=2
      settings: ActiveDisplayYMinimum=-2.7903298017751648  ActiveDisplayYMaximum=-1.7770998587100291  DataLoggingVariableName=ScopeData10
  "Sinusoidal Measurement (PLL, Three-Phase)" : eeSinusoidalMeasurementV2/Sinusoidal Measurement (PLL, Three-Phase)  InputFilter=on  InputNormalization=off  Kp_LF=40  Ki_LF=1000  F0=frequency  Theta0=0  Ts=Ts
  Terminator : Terminator
  Terminator1 : Terminator
  mag : Outport
  freq : Outport  Port=2
  angle : Outport  Port=3
  Vd : Outport  Port=4
  Vq : Outport  Port=5
  Id1 : Outport  Port=6
  Iq1 : Outport  Port=7
  wires:
  Iabc/1 -> Park Transform1/1
  Demux1/3 -> Terminator1/1
  Demux1/2 -> Scope1/2, Iq1/1
  Demux1/1 -> Scope1/1, Id1/1
  Park Transform1/1 -> Demux1/1
  "Sinusoidal Measurement (PLL, Three-Phase)"/3 -> mag/1
  "Sinusoidal Measurement (PLL, Three-Phase)"/1 -> freq/1
  "Sinusoidal Measurement (PLL, Three-Phase)"/2 -> Park Transform/2, Park Transform1/2, angle/1
  Demux/2 -> Vq/1, Scope/2
  Demux/1 -> Vd/1, Scope/1
  Park Transform/1 -> Demux/1
  Vabc/1 -> "Sinusoidal Measurement (PLL, Three-Phase)"/1, Park Transform/1
  Demux/3 -> Terminator/1

== system MicrogridControl/BESS/BESS Integrated1/Simplified/Grid Forming/Reference Generator/If Action Subsystem ==
  PRef : Inport
  P : Inport  Port=2
  QRef : Inport  Port=3
  Q : Inport  Port=4
  Action Port : ActionPort
  Add : Sum  Inputs=-+
  Add1 : Sum  Inputs=+-
  Add2 : Sum
  Add3 : Sum  Inputs=+-
  Add4 : Sum  Inputs=-+
  Constant : Constant  Value=2*pi*frequency  SampleTime=-1
  Constant2 : Constant
  Constant3 : Constant
  Gain : Gain  Gain=activeDroop
  Gain1 : Gain  Gain=reactiveDroop
  Gain4 : Gain  Gain=Vac
  Gain5 : Gain  Gain=2*pi*frequency
  Integrator with Wrapped State (Discrete or Continuous) : eeGeneralControl/Integrator with Wrapped State (Discrete or Continuous)  LabelModeActiveChoice=Discrete  WrappedStateUpperValue=2*pi  WrappedStateLowerValue=0  x0=0  Ts=-1
  Integrator with Wrapped State (Discrete or Continuous)1 : eeGeneralControl/Integrator with Wrapped State (Discrete or Continuous)  LabelModeActiveChoice=Discrete  WrappedStateUpperValue=2*pi  WrappedStateLowerValue=0  x0=0  Ts=-1
  Saturation : Saturate  UpperLimit=1.1  LowerLimit=0.9
  Scope : Scope
      settings: ActiveDisplayYMinimum=-1  ActiveDisplayYMaximum=1  DataLoggingVariableName=ScopeData2
  Scope1 : Scope
      settings: ActiveDisplayYMinimum=-1  ActiveDisplayYMaximum=1  DataLoggingVariableName=ScopeData3
  Scope2 : Scope  NumInputPorts=2
      settings: ActiveDisplayYMinimum=-1  ActiveDisplayYMaximum=1
  Scope3 : Scope  NumInputPorts=2
      settings: ActiveDisplayYMinimum=-1  ActiveDisplayYMaximum=1  DataLoggingVariableName=ScopeData2
  Vt : Outport
  Ph : Outport  Port=2
  wires:
  Add4/1 -> Scope/1, Gain5/1
  Gain/1 -> Add4/1
  Add1/1 -> Gain1/1
  Add2/1 -> Scope1/1, Saturation/1
  Gain5/1 -> Integrator with Wrapped State (Discrete or Continuous)/1
  Constant3/1 -> Add4/2
  Integrator with Wrapped State (Discrete or Continuous)/1 -> Add3/1
  Constant2/1 -> Add2/2
  Gain1/1 -> Add2/1
  Gain4/1 -> Vt/1
  QRef/1 -> Add1/1, Scope2/1
  Saturation/1 -> Gain4/1
  Add/1 -> Gain/1
  PRef/1 -> Add/1, Scope3/1
  Add3/1 -> Ph/1
  Constant/1 -> Integrator with Wrapped State (Discrete or Continuous)1/1
  Integrator with Wrapped State (Discrete or Continuous)1/1 -> Add3/2
  P/1 -> Add/2, Scope3/2
  Q/1 -> Add1/2, Scope2/2

== system MicrogridControl/BESS/BESS Integrated1/Simplified/Grid Forming/Reference Generator/If Action Subsystem1 ==
  PRef : Inport
  P : Inport  Port=2
  VRef : Inport  Port=3
  V : Inport  Port=4
  Action Port : ActionPort
  Add : Sum  Inputs=+-
  Add1 : Sum  Inputs=+-
  Add2 : Sum
  Add3 : Sum  Inputs=+-
  Add4 : Sum  Inputs=-+
  Constant2 : Constant
  Constant3 : Constant
  Constant4 : Constant  Value=0
  Gain : Gain  Gain=reactiveDroop
  Gain1 : Gain  Gain=activeDroop
  Gain4 : Gain  Gain=systemVoltage
  Gain5 : Gain  Gain=2*pi*systemFrequency
  Integrator with Wrapped State (Discrete or Continuous) : eeGeneralControl/Integrator with Wrapped State (Discrete or Continuous)  LabelModeActiveChoice=Discrete  WrappedStateUpperValue=2*pi  WrappedStateLowerValue=0  x0=0  Ts=-1
  Saturation : Saturate  UpperLimit=1.1  LowerLimit=0.9
  Vt : Outport
  Ph : Outport  Port=2
  wires:
  Add/1 -> Gain/1
  Constant4/1 -> Add3/2
  Add4/1 -> Gain5/1
  Gain/1 -> Add4/1
  Add1/1 -> Gain1/1
  Add2/1 -> Saturation/1
  Gain5/1 -> Integrator with Wrapped State (Discrete or Continuous)/1
  Constant3/1 -> Add4/2
  Integrator with Wrapped State (Discrete or Continuous)/1 -> Add3/1
  Constant2/1 -> Add2/2
  Gain1/1 -> Add2/1
  V/1 -> Add/2
  Gain4/1 -> Vt/1
  P/1 -> Add1/2
  VRef/1 -> Add/1
  PRef/1 -> Add1/1
  Add3/1 -> Ph/1
  Saturation/1 -> Gain4/1
